simulink model "AVS_SIM4"  (R2020a)
settings: Solver=VariableStepAuto  StartTime=0.0  StopTime=25000  RelTol=1e-3
undefined symbols (not defined in the file): a, b
settings Model: Creator=Jaka  LastModifiedBy=Jaka

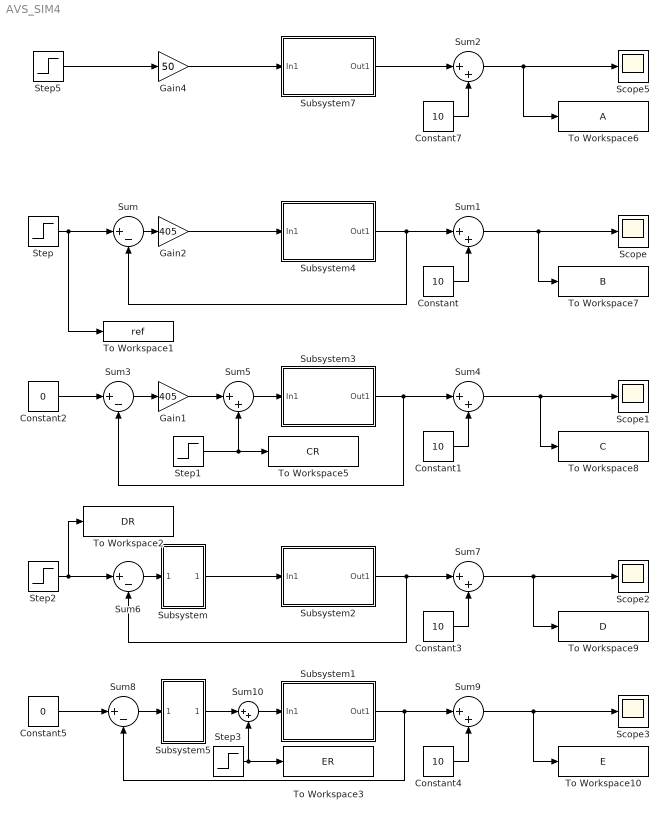
== system AVS_SIM4 ==
  Constant{,1,3..4,7} (5 alike) : Constant  Value=10
  Constant2 : Constant  Value=0
  Constant5 : Constant  Value=0
  Gain1 : Gain  Gain=405
  Gain2 : Gain  Gain=405
  Gain4 : Gain  Gain=50
  Scope{,1..3,5} (5 alike) : Scope
  Step : Step  Time=10000  After=10  SampleTime=0
  Step1 : Step  Time=10000  After=250  SampleTime=0
  Step2 : Step  Time=10000  After=10  SampleTime=0
  Step3 : Step  Time=10000  After=250  SampleTime=0
  Step5 : Step  Time=10000  After=10  SampleTime=0
  Subsystem : Subsystem
  Subsystem1 : Subsystem
  Subsystem2 : Subsystem
  Subsystem3 : Subsystem
  Subsystem4 : Subsystem
  Subsystem5 : Subsystem
  Subsystem7 : Subsystem
  Sum{,3,6,8} (4 alike) : Sum  Inputs=|+-
  Sum{1..2,4..5,7,9..10} (7 alike) : Sum  Inputs=|++
  To Workspace1 : ToWorkspace  VariableName=ref  SampleTime=-1
  To Workspace10 : ToWorkspace  VariableName=E  SampleTime=-1
  To Workspace2 : ToWorkspace  VariableName=DR  SampleTime=-1
  To Workspace3 : ToWorkspace  VariableName=ER  SampleTime=-1
  To Workspace5 : ToWorkspace  VariableName=CR  SaveFormat=Timeseries  SampleTime=1
  To Workspace6 : ToWorkspace  VariableName=A  SampleTime=-1
  To Workspace7 : ToWorkspace  VariableName=B  SampleTime=-1
  To Workspace8 : ToWorkspace  VariableName=C  SampleTime=-1
  To Workspace9 : ToWorkspace  VariableName=D  SampleTime=-1
  wires:
  Step5/1 -> Gain4/1
  Subsystem4/1(Out1) -> Sum1/1, Sum/2
  Sum4/1 -> To Workspace8/1, Scope1/1
  Constant5/1 -> Sum8/1
  Subsystem5/1(Out1) -> Sum10/1
  Subsystem7/1(Out1) -> Sum2/1
  Gain4/1 -> Subsystem7/1(In1)
  Sum2/1 -> To Workspace6/1, Scope5/1
  Constant7/1 -> Sum2/2
  Subsystem3/1(Out1) -> Sum4/1, Sum3/2
  Sum9/1 -> To Workspace10/1, Scope3/1
  Constant3/1 -> Sum7/2
  Sum8/1 -> Subsystem5/1(In1)
  Sum3/1 -> Gain1/1
  Sum6/1 -> Subsystem/1(In1)
  Constant1/1 -> Sum4/2
  Sum5/1 -> Subsystem3/1(In1)
  Constant2/1 -> Sum3/1
  Step2/1 -> To Workspace2/1, Sum6/1
  Sum7/1 -> To Workspace9/1, Scope2/1
  Step3/1 -> To Workspace3/1, Sum10/2
  Constant4/1 -> Sum9/2
  Subsystem1/1(Out1) -> Sum9/1, Sum8/2
  Subsystem2/1(Out1) -> Sum7/1, Sum6/2
  Sum10/1 -> Subsystem1/1(In1)
  Subsystem/1(Out1) -> Subsystem2/1(In1)
  Gain1/1 -> Sum5/1
  Step1/1 -> Sum5/2, To Workspace5/1
  Constant/1 -> Sum1/2
  Sum/1 -> Gain2/1
  Sum1/1 -> To Workspace7/1, Scope/1
  Gain2/1 -> Subsystem4/1(In1)
  Step/1 -> To Workspace1/1, Sum/1

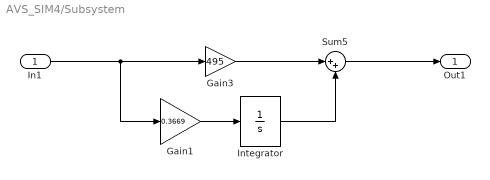
== system AVS_SIM4/Subsystem ==
  In1 : Inport
  Gain1 : Gain  Gain=0.3669
  Gain3 : Gain  Gain=495
  Integrator : Integrator
  Sum5 : Sum  Inputs=|++
  Out1 : Outport
  wires:
  In1/1 -> Gain3/1, Gain1/1
  Gain1/1 -> Integrator/1
  Integrator/1 -> Sum5/2
  Gain3/1 -> Sum5/1
  Sum5/1 -> Out1/1

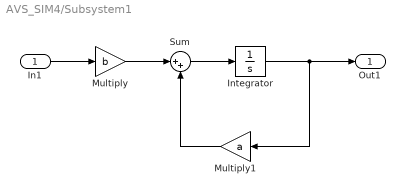
== system AVS_SIM4/Subsystem1 ==
  In1 : Inport
  Integrator : Integrator  InitialCondition=-5
  Multiply : Gain  Gain=b
  Multiply1 : Gain  Gain=a
  Sum : Sum  Inputs=|++
  Out1 : Outport
  wires:
  Multiply1/1 -> Sum/2
  Sum/1 -> Integrator/1
  In1/1 -> Multiply/1
  Multiply/1 -> Sum/1
  Integrator/1 -> Out1/1, Multiply1/1

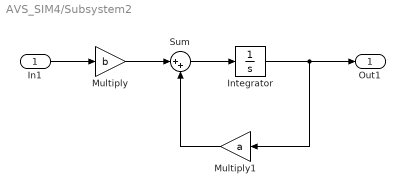
== system AVS_SIM4/Subsystem2 ==
  In1 : Inport
  Integrator : Integrator  InitialCondition=-5
  Multiply : Gain  Gain=b
  Multiply1 : Gain  Gain=a
  Sum : Sum  Inputs=|++
  Out1 : Outport
  wires:
  Multiply1/1 -> Sum/2
  Sum/1 -> Integrator/1
  In1/1 -> Multiply/1
  Multiply/1 -> Sum/1
  Integrator/1 -> Out1/1, Multiply1/1

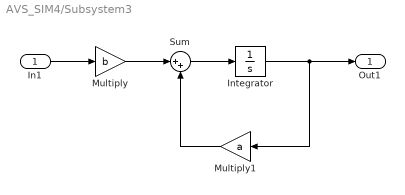
== system AVS_SIM4/Subsystem3 ==
  In1 : Inport
  Integrator : Integrator  InitialCondition=-5
  Multiply : Gain  Gain=b
  Multiply1 : Gain  Gain=a
  Sum : Sum  Inputs=|++
  Out1 : Outport
  wires:
  Multiply1/1 -> Sum/2
  Sum/1 -> Integrator/1
  In1/1 -> Multiply/1
  Multiply/1 -> Sum/1
  Integrator/1 -> Out1/1, Multiply1/1

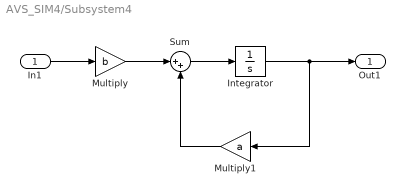
== system AVS_SIM4/Subsystem4 ==
  In1 : Inport
  Integrator : Integrator  InitialCondition=-5
  Multiply : Gain  Gain=b
  Multiply1 : Gain  Gain=a
  Sum : Sum  Inputs=|++
  Out1 : Outport
  wires:
  Multiply1/1 -> Sum/2
  Sum/1 -> Integrator/1
  In1/1 -> Multiply/1
  Multiply/1 -> Sum/1
  Integrator/1 -> Out1/1, Multiply1/1

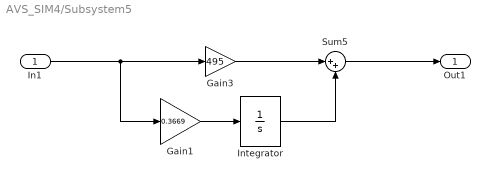
== system AVS_SIM4/Subsystem5 ==
  In1 : Inport
  Gain1 : Gain  Gain=0.3669
  Gain3 : Gain  Gain=495
  Integrator : Integrator
  Sum5 : Sum  Inputs=|++
  Out1 : Outport
  wires:
  In1/1 -> Gain3/1, Gain1/1
  Gain1/1 -> Integrator/1
  Integrator/1 -> Sum5/2
  Gain3/1 -> Sum5/1
  Sum5/1 -> Out1/1

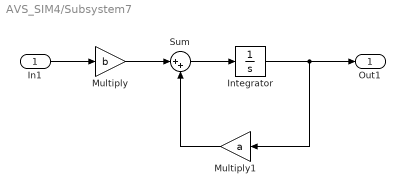
== system AVS_SIM4/Subsystem7 ==
  In1 : Inport
  Integrator : Integrator  InitialCondition=-5
  Multiply : Gain  Gain=b
  Multiply1 : Gain  Gain=a
  Sum : Sum  Inputs=|++
  Out1 : Outport
  wires:
  Multiply1/1 -> Sum/2
  Sum/1 -> Integrator/1
  In1/1 -> Multiply/1
  Multiply/1 -> Sum/1
  Integrator/1 -> Out1/1, Multiply1/1
